simulink model "logger_task"  (Simulink 3.00)
libraries: arclib x2, mathlib x1

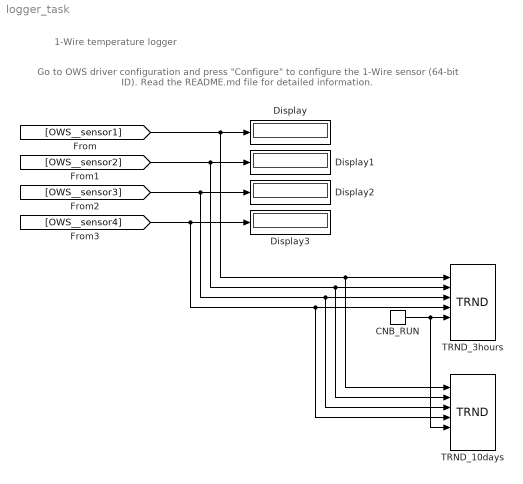
== system logger_task ==
  note: 1-Wire temperature logger
  note: Go to OWS driver configuration and press "Configure" to configure the 1-Wire sensor (64-bit ID).
      |
      | Read the README.md file for detailed information.
  CNB_RUN : mathlib/CNB  SystemSampleTime=-1  YCN=on
  Display{,1..3} (4 alike) : Display
      settings: Format=Best fit  Suffix=°C
  TRND_10days : arclib/TRND  SystemSampleTime=-1  n=4  l=86400  btype=8: Double  ptype1=1: Store  ptype2=1: Store  ptype3=1: Store  ptype4=1: Store  pfac=20  afac=0  arc=0  id=2  Title=Temperatures (10 days)  timesrc=1
  TRND_3hours : arclib/TRND  SystemSampleTime=-1  n=4  l=5400  btype=8: Double  ptype1=1: Store  ptype2=1: Store  ptype3=1: Store  ptype4=1: Store  pfac=4  afac=0  arc=0  id=1  Title=Temperatures (3 hours)  timesrc=1
  wires:
  CNB_RUN/1 -> TRND_10days/5, TRND_3hours/5
  [OWS__sensor1] -> TRND_10days/1, TRND_3hours/1, Display/1
  [OWS__sensor2] -> TRND_10days/2, TRND_3hours/2, Display1/1
  [OWS__sensor3] -> TRND_10days/3, TRND_3hours/3, Display2/1
  [OWS__sensor4] -> TRND_10days/4, TRND_3hours/4, Display3/1
